simulink library "simeventsattributes2"  (Simulink 7.1)
undefined symbols (not defined in the file or in its folder): des_support, gcbh
libraries: des_sfun_lib x1, simeventsattributes1 x1
settings Model: Creator=mclune  LastModifiedBy=ywu  ExtModeAutoUpdateStatusClock=off

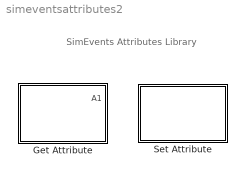
== system simeventsattributes2 ==
  note: SimEvents Attributes Library
  Get Attribute : Subsystem  Priority=1  DialogController=des_ddg_create  DialogControllerArgs=DataTag1  LoadFcn=des_support('desLoadFcn',gcbh)  StartFcn=des_support('desStartFcn',gcbh)  StopFcn=des_support('desStopFcn',gcbh)  mask(Get Attribute){AttributeName=Attribute1, AttributeMissing=Error, AttributeDefaultValue=1, AttributeSendTiming=After entity departure, AttributeTreatAsVector=1, StatNumberDeparted=Off, EvaluatedDefaultAttributeValue={[]}}
      mask prompts: AttributeName "Attribute name:"; AttributeMissing "Action for missing attribute:"; AttributeDefaultValue "Default value:"; AttributeSendTiming "Send attribute value:"; AttributeTreatAsVector "Treat vector as 1-D:"; StatNumberDeparted "Number of entities departed, #d:"; EvaluatedDefaultAttributeValue "DefaultValue for Evaluation"
      mask help: Output attribute values to signal ports for each departing entity.
      mask init:
      | AttributeTable = des_ddg_init(gcbh,'GetAttribute');
      settings: CopyFcn=des_support('desCopyFcn',gcbh)  DeleteFcn=des_support('desDeleteFcn',gcbh)  UndoDeleteFcn=des_support('desUndoDeleteFcn',gcbh)  ModelCloseFcn=des_support('desModelCloseFcn',gcbh)  PreSaveFcn=des_support('desPreSaveFcn',gcbh)  PostSaveFcn=des_support('desPostSaveFcn',gcbh)  NameChangeFcn=des_support('desNameChangeFcn',gcbh)  CloseFcn=des_support('desCloseFcn',gcbh)  ErrorFcn=des_error_redirect
      mask Help: helpview(simeventsbhelp)
      mask StyleString: edit,edit,edit,edit,edit,popup(Off|On|Upon stop or pause),edit
      mask CallbackString: ||des_setEvaluatedAttributes(gcb,'GetAttribute');||||
      mask TabNameString: A1,A1,A1,A1,A1,Statistics,Statistics
      mask Display:
      | image(des_iconLoad('attrGet.jpg'),'center');
      | port_label('LConn',1,'IN');
      | port_label('output',1,'A1');
      | port_label('RConn',1,'OUT');
  Set Attribute : Subsystem  Priority=1  DialogController=des_ddg_create  DialogControllerArgs=DataTag4  LoadFcn=des_support('desLoadFcn',gcbh)  StartFcn=des_support('desStartFcn',gcbh)  StopFcn=des_support('desStopFcn',gcbh)  mask(Set Attribute){AttributeFrom=Dialog, AttributeName=Attribute1, AttributeTreatAsVector=1, AttributeValue=1, AttributeCreate=on, StatNumberDeparted=Off, EvaluatedAttributeValue={1}}
      mask prompts: AttributeFrom "Attribute assignment:"; AttributeName "Attribute name:"; AttributeTreatAsVector "Type:"; AttributeValue "Value:"; AttributeCreate "Create attribute if not present"; StatNumberDeparted "Number of entities departed, #d:"; EvaluatedAttributeValue "Attribute Value for Evaluation"
      mask help: Set attribute values using data from the dialog or signals for each departing entity.
      mask init:
      | AttributeTable = des_ddg_init(gcbh,'SetAttribute');
      settings: CopyFcn=des_support('desCopyFcn',gcbh)  DeleteFcn=des_support('desDeleteFcn',gcbh)  UndoDeleteFcn=des_support('desUndoDeleteFcn',gcbh)  ModelCloseFcn=des_support('desModelCloseFcn',gcbh)  PreSaveFcn=des_support('desPreSaveFcn',gcbh)  PostSaveFcn=des_support('desPostSaveFcn',gcbh)  NameChangeFcn=des_support('desNameChangeFcn',gcbh)  CloseFcn=des_support('desCloseFcn',gcbh)  ErrorFcn=des_error_redirect
      mask Help: helpview(simeventsbhelp)
      mask StyleString: edit,edit,edit,edit,checkbox,popup(Off|On|Upon stop or pause),edit
      mask CallbackString: |||des_setEvaluatedAttributes(gcb,'SetAttribute');|||
      mask TabNameString: A1,A1,A1,A1,A1,Statistics,Statistics
      mask Display:
      | image(des_iconLoad('attrSet.jpg'),'center');
      | port_label('LConn',1,'IN');
      | port_label('RConn',1,'OUT');

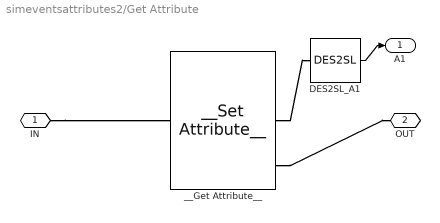
== system simeventsattributes2/Get Attribute ==
  DES2SL_A1 : des_sfun_lib/DES2SL  SystemSampleTime=-1  PortType=desPortIn  PhysicalDomain=simevents  SubClassName=DES_DES2SL  timingControl=SimEvents  execIndex=0  multipleOutputs=off  updateBeforeRead=off  InitValue=0  sampleTime=-1  offsetTime=0  idxBlockMR=0  IsMonitorOnly=off  dimsInfo=-1
  __Get Attribute__ : simeventsattributes1/Set Attribute/__Set Attribute__  PhysicalDomain=simevents  SubClassName=DES_GETATTRIBUTEV2  LeftPortType=desPortIn  RightPortType=desPortOut  LConnTagsString=DI  RConnTagsString=DO|DO|DO
  IN : PMIOPort  Port=1  Side=Left
  OUT : PMIOPort  Orientation=left  Port=2  Side=Right
  A1 : Outport  OutDataType=sfix(16)  OutScaling=2^0
  wires:
  DES2SL_A1/1 -> A1/1
  connections:
  IN/RConn1 -- __Get Attribute__/LConn1
  __Get Attribute__/RConn3 -- OUT/RConn1
  __Get Attribute__/RConn2 -- DES2SL_A1/LConn1

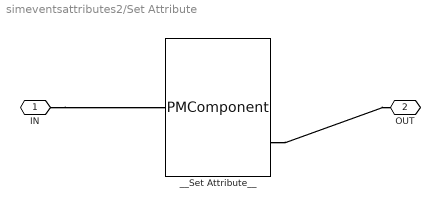
== system simeventsattributes2/Set Attribute ==
  __Set Attribute__ : PMComponent  PhysicalDomain=simevents  SubClassName=DES_SETATTRIBUTEV2  LeftPortType=desPortIn  RightPortType=desPortOut  LConnTagsString=DI  RConnTagsString=DO|DO
      mask Display:
      | port_label('LConn',1,'IN');
      | port_label('RConn',1,'#d');
      | port_label('RConn',2,'OUT');
  IN : PMIOPort  Port=1  Side=Left
  OUT : PMIOPort  Orientation=left  Port=2  Side=Right
  connections:
  IN/RConn1 -- __Set Attribute__/LConn1
  __Set Attribute__/RConn2 -- OUT/RConn1
